simulink model "TADPOLE_Closed_Loop_v2"  (R2024b)
settings: Solver=VariableStepAuto  StartTime=0.0  StopTime=19  RelTol=1e-3
InitFcn:
  | clear mex;
values from neighbouring files (symbols this model uses):
  ipa_tank = 700    [TADPOLEControl.m]
  ox_tank = 600    [TADPOLEControl.m]
  timeDelta = 1/5000    (= 0.0002)    [TADPOLEControl.m]
  timeDeltaCMD = 1/1000    (= 0.001)    [TADPOLEControl.m]
  timeDeltaOUT = 1/200    (= 0.005)    [TADPOLEControl.m]
  x0 = [0 0 0 0]    [TADPOLEControl.m]
undefined symbols (not defined in the file or in its folder): DiscIntNeverNeededParam
settings Model: Creator=pplat  LastModifiedBy=pplat
settings DebuggingCC: AlgebraicLoopMsg=none

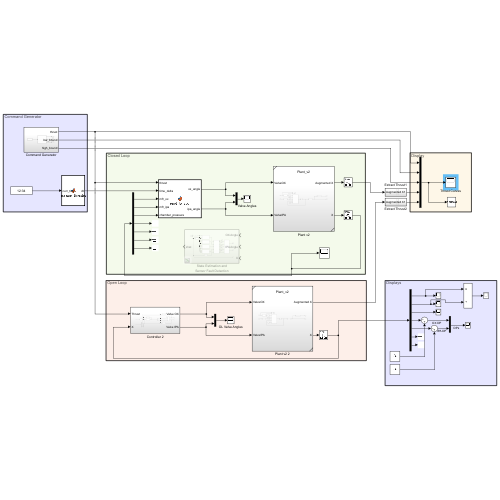
[thumbnail: Simulink's stored preview of the top-level diagram]
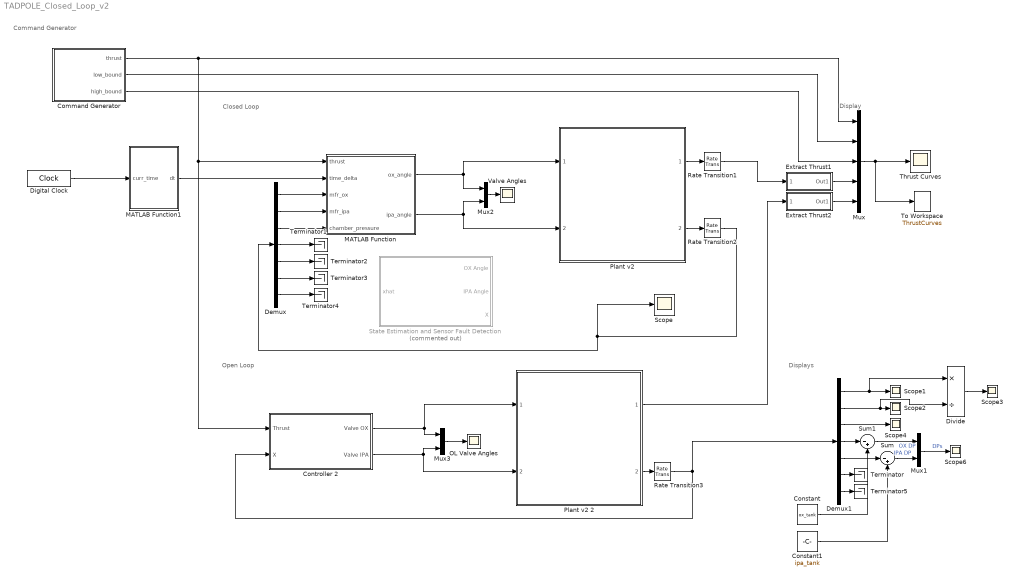
== system TADPOLE_Closed_Loop_v2 ==
  note: Displays
  note: Display
  note: Open Loop
  note: Closed Loop
  note: Command Generator
  Command Generator : Subsystem
  Constant : Constant  Value=ox_tank
  Constant1 : Constant  Value=ipa_tank
  Controller 2 : Subsystem
  Demux : Demux  Outputs=7
  Demux1 : Demux  Outputs=7
  Digital Clock : DigitalClock  SampleTime=timeDelta
  Divide : Product  Inputs=*/
  Extract Thrust1 : Subsystem
  Extract Thrust2 : Subsystem
  MATLAB Function : MATLAB Function  TreatAsAtomicUnit=on
  MATLAB Function1 : MATLAB Function  TreatAsAtomicUnit=on
  Mux : Mux  Inputs=5
  Mux1 : Mux  Inputs=2
  Mux2 : Mux  Inputs=2
  Mux3 : Mux  Inputs=2
  OL Valve Angles : Scope
  Plant v2 : Subsystem  ReferencedSubsystem=Plant_v2
  Plant v2 2 : Subsystem  ReferencedSubsystem=Plant_v2
  Rate Transition1 : RateTransition  OutPortSampleTime=timeDeltaOUT
  Rate Transition2 : RateTransition  OutPortSampleTime=timeDeltaOUT
  Rate Transition3 : RateTransition  OutPortSampleTime=timeDeltaOUT
  Scope{,1..4,6} (6 alike) : Scope
  State Estimation and Sensor Fault Detection : Subsystem  Commented=on
  Sum : Sum  Inputs=|-+
  Sum1 : Sum  Inputs=|-+
  Terminator{,1..5} (6 alike) : Terminator
  Thrust Curves : Scope
  To Workspace : ToWorkspace  VariableName=ThrustCurves  SaveFormat=Timeseries  SampleTime=-1
  Valve Angles : Scope
  wires:
  Mux/1 -> To Workspace/1, Thrust Curves/1
  Mux2/1 -> Valve Angles/1
  Command Generator/1(thrust) -> Mux/1, Controller 2/1(Thrust), MATLAB Function/1(thrust)
  Command Generator/2(low_bound) -> Mux/2
  Command Generator/3(high_bound) -> Mux/3
  MATLAB Function1/1(dt) -> MATLAB Function/2(time_delta)
  Mux3/1 -> OL Valve Angles/1
  Digital Clock/1 -> MATLAB Function1/1(curr_time)
  MATLAB Function/1(ox_angle) -> Mux2/1, Plant v2/1
  MATLAB Function/2(ipa_angle) -> Plant v2/2, Mux2/2
  Controller 2/1(Valve OX) -> Plant v2 2/1, Mux3/1
  Controller 2/2(Valve IPA) -> Plant v2 2/2, Mux3/2
  Extract Thrust1/1(Out1) -> Mux/4
  Extract Thrust2/1(Out1) -> Mux/5
  Plant v2/1 -> Rate Transition1/1
  Plant v2 2/1 -> Extract Thrust2/1(Augmented X)
  Rate Transition1/1 -> Extract Thrust1/1(Augmented X)
  Plant v2/2 -> Rate Transition2/1
  Demux/3 -> MATLAB Function/5(chamber_pressure)
  Demux/2 -> MATLAB Function/4(mfr_ipa)
  Demux/1 -> MATLAB Function/3(mfr_ox)
  Demux/4 -> Terminator1/1
  Demux/5 -> Terminator2/1
  Rate Transition2/1 -> Scope/1, Demux/1
  Demux/6 -> Terminator3/1
  Demux/7 -> Terminator4/1
  Sum1/1 -> Mux1/1  "OX DP"
  Demux1/3 -> Scope4/1
  Divide/1 -> Scope3/1
  Demux1/2 -> Divide/2, Scope2/1
  Mux1/1 -> Scope6/1  "DPs"
  Plant v2 2/2 -> Rate Transition3/1
  Demux1/4 -> Sum1/1
  Demux1/1 -> Divide/1, Scope1/1
  Demux1/5 -> Sum/1
  Constant/1 -> Sum1/2
  Constant1/1 -> Sum/2
  Sum/1 -> Mux1/2  "IPA DP"
  Demux1/6 -> Terminator/1
  Demux1/7 -> Terminator5/1
  Rate Transition3/1 -> Controller 2/2(X), Demux1/1

== system TADPOLE_Closed_Loop_v2/Command Generator ==
  Digital Clock : DigitalClock  SampleTime=timeDelta
  MATLAB Function : MATLAB Function  TreatAsAtomicUnit=on
  thrust : Outport
  low_bound : Outport  Port=2
  high_bound : Outport  Port=3
  wires:
  MATLAB Function/1(thrust) -> thrust/1
  Digital Clock/1 -> MATLAB Function/1(time)
  MATLAB Function/2(low_bound) -> low_bound/1
  MATLAB Function/3(high_bound) -> high_bound/1

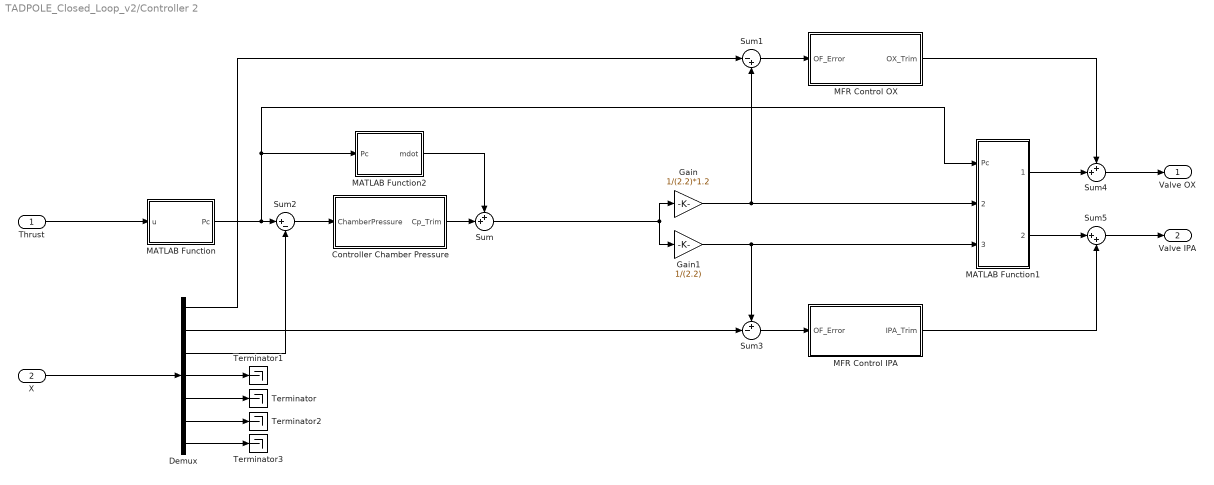
== system TADPOLE_Closed_Loop_v2/Controller 2 ==
  Thrust : Inport
  X : Inport  Port=2
  Controller Chamber Pressure : Subsystem
      settings: PortSchema="{\"entries\":[{\"content\":{\"sides\":[{\"content\":{\"connectorIds\":[\"Out1\"]},\"type\":\"ConnectorPlacement.EquallySpacedRectSide\",\"uuid\":\"33f68c87-1ae2-45d4-8ad9-4cf3c5bc8584\"},{\"content\":{\"connectorIds\":[\"In1\"],\"side\":\"RIGHT\"},\"type\":\"ConnectorPlacement.EquallySpacedRectSide\",\"uuid\":\"17976ab6-0faa-4d7d-91ba-f8a21a62dc32\"},{\"content\":{\"side\":\"TOP\"},\"type\":\"ConnectorPlacement.EquallySpacedRectSide\",\"uuid\":\"89a256ba-7dd2-41f4-a68b-27cc674e20da\"},{\"content\":{\"side\":\"BOTTOM\"},\"type\":\"ConnectorPlacement.EquallySpacedRectSide\",\"uuid\":\"73e60893-e40b-4ea1-8c2d-1d944b0843d3\"}]},\"type\":\"ConnectorPlacement.EquallySpacedConnector\",\"uuid\":\"c17bed4f-f3ae-43fd-abcb-ba9ac56db614\"}],\"packageUris\":[\"http://schema.mathworks.com/mf0/Connector/R2020b\"],\"version\":\"1.0\"}"
  Demux : Demux  Outputs=7
  Gain : Gain  Gain=1/(2.2)*1.2
  Gain1 : Gain  Gain=1/(2.2)
  MATLAB Function : MATLAB Function  TreatAsAtomicUnit=on
  MATLAB Function1 : MATLAB Function  TreatAsAtomicUnit=on
  MATLAB Function2 : MATLAB Function  TreatAsAtomicUnit=on
  MFR Control IPA : Subsystem
      settings: PortSchema="{\"entries\":[{\"content\":{\"sides\":[{\"content\":{\"connectorIds\":[\"Out1\"]},\"type\":\"ConnectorPlacement.EquallySpacedRectSide\",\"uuid\":\"33f68c87-1ae2-45d4-8ad9-4cf3c5bc8584\"},{\"content\":{\"connectorIds\":[\"In1\"],\"side\":\"RIGHT\"},\"type\":\"ConnectorPlacement.EquallySpacedRectSide\",\"uuid\":\"17976ab6-0faa-4d7d-91ba-f8a21a62dc32\"},{\"content\":{\"side\":\"TOP\"},\"type\":\"ConnectorPlacement.EquallySpacedRectSide\",\"uuid\":\"89a256ba-7dd2-41f4-a68b-27cc674e20da\"},{\"content\":{\"side\":\"BOTTOM\"},\"type\":\"ConnectorPlacement.EquallySpacedRectSide\",\"uuid\":\"73e60893-e40b-4ea1-8c2d-1d944b0843d3\"}]},\"type\":\"ConnectorPlacement.EquallySpacedConnector\",\"uuid\":\"c17bed4f-f3ae-43fd-abcb-ba9ac56db614\"}],\"packageUris\":[\"http://schema.mathworks.com/mf0/Connector/R2020b\"],\"version\":\"1.0\"}"
  MFR Control OX : Subsystem
      settings: PortSchema="{\"entries\":[{\"content\":{\"sides\":[{\"content\":{\"connectorIds\":[\"Out1\"]},\"type\":\"ConnectorPlacement.EquallySpacedRectSide\",\"uuid\":\"33f68c87-1ae2-45d4-8ad9-4cf3c5bc8584\"},{\"content\":{\"connectorIds\":[\"In1\"],\"side\":\"RIGHT\"},\"type\":\"ConnectorPlacement.EquallySpacedRectSide\",\"uuid\":\"17976ab6-0faa-4d7d-91ba-f8a21a62dc32\"},{\"content\":{\"side\":\"TOP\"},\"type\":\"ConnectorPlacement.EquallySpacedRectSide\",\"uuid\":\"89a256ba-7dd2-41f4-a68b-27cc674e20da\"},{\"content\":{\"side\":\"BOTTOM\"},\"type\":\"ConnectorPlacement.EquallySpacedRectSide\",\"uuid\":\"73e60893-e40b-4ea1-8c2d-1d944b0843d3\"}]},\"type\":\"ConnectorPlacement.EquallySpacedConnector\",\"uuid\":\"c17bed4f-f3ae-43fd-abcb-ba9ac56db614\"}],\"packageUris\":[\"http://schema.mathworks.com/mf0/Connector/R2020b\"],\"version\":\"1.0\"}"
  Sum : Sum  Inputs=++|
  Sum1 : Sum  Inputs=|-+
  Sum2 : Sum  Inputs=|+-
  Sum3 : Sum  Inputs=+-|
  Sum4 : Sum  Inputs=++|
  Sum5 : Sum  Inputs=|++
  Terminator{,1..3} (4 alike) : Terminator
  Valve OX : Outport
  Valve IPA : Outport  Port=2
  wires:
  MATLAB Function/1(Pc) -> MATLAB Function2/1(Pc), MATLAB Function1/1(Pc), Sum2/1
  MATLAB Function2/1(mdot) -> Sum/1
  Sum2/1 -> Controller Chamber Pressure/1(ChamberPressure)
  Controller Chamber Pressure/1(Cp_Trim) -> Sum/2
  Demux/1 -> Sum1/1
  Demux/2 -> Sum3/2
  Sum3/1 -> MFR Control IPA/1(OF_Error)
  Sum1/1 -> MFR Control OX/1(OF_Error)
  Thrust/1 -> MATLAB Function/1(u)
  Sum/1 -> Gain/1, Gain1/1
  Gain/1 -> Sum1/2, MATLAB Function1/2(mdot_ox)
  Gain1/1 -> MATLAB Function1/3(mdot_ipa), Sum3/1
  X/1 -> Demux/1
  Demux/5 -> Terminator/1
  Demux/4 -> Terminator1/1
  Demux/3 -> Sum2/2
  Sum5/1 -> Valve IPA/1
  MATLAB Function1/2(theta_ipa) -> Sum5/1
  MATLAB Function1/1(theta_ox) -> Sum4/2
  Sum4/1 -> Valve OX/1
  MFR Control OX/1(OX_Trim) -> Sum4/1
  MFR Control IPA/1(IPA_Trim) -> Sum5/2
  Demux/6 -> Terminator2/1
  Demux/7 -> Terminator3/1

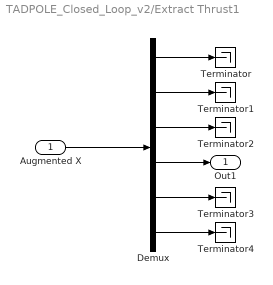
== system TADPOLE_Closed_Loop_v2/Extract Thrust1 ==
  Augmented X : Inport
  Demux : Demux  Outputs=6
  Terminator{,1..4} (5 alike) : Terminator
  Out1 : Outport
  wires:
  Augmented X/1 -> Demux/1
  Demux/1 -> Terminator/1
  Demux/2 -> Terminator1/1
  Demux/3 -> Terminator2/1
  Demux/5 -> Terminator3/1
  Demux/6 -> Terminator4/1
  Demux/4 -> Out1/1

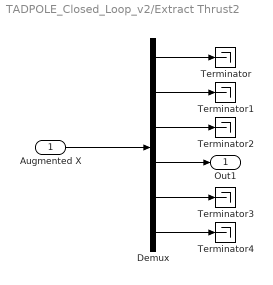
== system TADPOLE_Closed_Loop_v2/Extract Thrust2 ==
  Augmented X : Inport
  Demux : Demux  Outputs=6
  Terminator{,1..4} (5 alike) : Terminator
  Out1 : Outport
  wires:
  Augmented X/1 -> Demux/1
  Demux/1 -> Terminator/1
  Demux/2 -> Terminator1/1
  Demux/3 -> Terminator2/1
  Demux/5 -> Terminator3/1
  Demux/6 -> Terminator4/1
  Demux/4 -> Out1/1

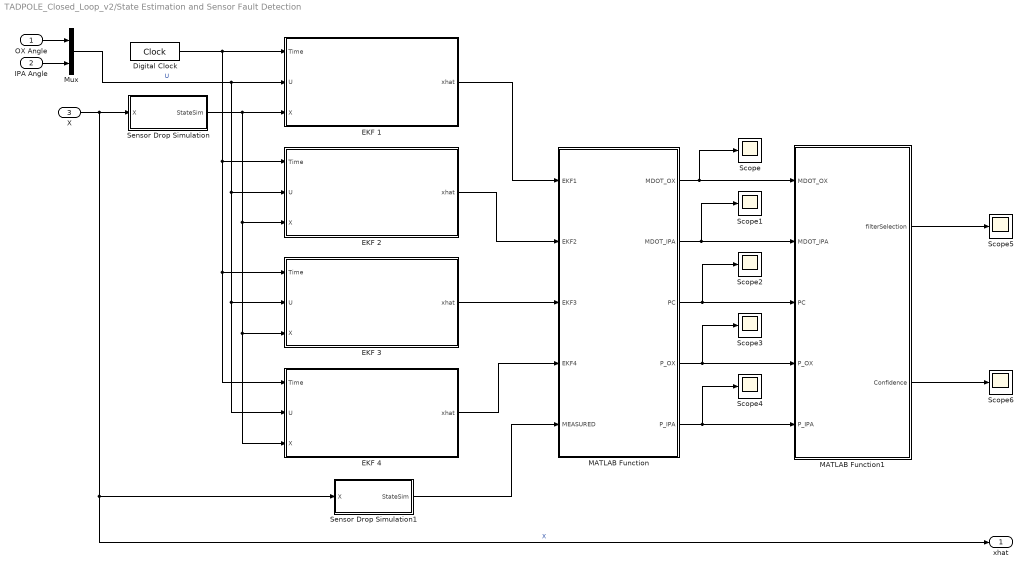
== system TADPOLE_Closed_Loop_v2/State Estimation and Sensor Fault Detection ==
  OX Angle : Inport
  IPA Angle : Inport  Port=2
  X : Inport  Port=3
  Digital Clock : DigitalClock  SampleTime=timeDeltaOUT
  EKF 1 : Subsystem
  EKF 2 : Subsystem
  EKF 3 : Subsystem
  EKF 4 : Subsystem
  MATLAB Function : MATLAB Function  TreatAsAtomicUnit=on
  MATLAB Function1 : MATLAB Function  TreatAsAtomicUnit=on
  Mux : Mux  Inputs=2
  Scope{,1..6} (7 alike) : Scope
  Sensor Drop Simulation : Subsystem
  Sensor Drop Simulation1 : Subsystem
  xhat : Outport
  wires:
  IPA Angle/1 -> Mux/2
  OX Angle/1 -> Mux/1
  X/1 -> Sensor Drop Simulation/1(X), xhat/1, Sensor Drop Simulation1/1(X)  "X"
  Mux/1 -> EKF 3/2(U), EKF 4/2(U), EKF 2/2(U), EKF 1/2(U)  "U"
  Digital Clock/1 -> EKF 3/1(Time), EKF 4/1(Time), EKF 2/1(Time), EKF 1/1(Time)
  Sensor Drop Simulation/1(StateSim) -> EKF 2/3(X), EKF 3/3(X), EKF 4/3(X), EKF 1/3(X)
  EKF 1/1(xhat) -> MATLAB Function/1(EKF1)
  EKF 2/1(xhat) -> MATLAB Function/2(EKF2)
  EKF 3/1(xhat) -> MATLAB Function/3(EKF3)
  EKF 4/1(xhat) -> MATLAB Function/4(EKF4)
  Sensor Drop Simulation1/1(StateSim) -> MATLAB Function/5(MEASURED)
  MATLAB Function/5(P_IPA) -> MATLAB Function1/5(P_IPA), Scope4/1
  MATLAB Function/4(P_OX) -> MATLAB Function1/4(P_OX), Scope3/1
  MATLAB Function/3(PC) -> Scope2/1, MATLAB Function1/3(PC)
  MATLAB Function/2(MDOT_IPA) -> MATLAB Function1/2(MDOT_IPA), Scope1/1
  MATLAB Function/1(MDOT_OX) -> Scope/1, MATLAB Function1/1(MDOT_OX)
  MATLAB Function1/1(filterSelection) -> Scope5/1
  MATLAB Function1/2(Confidence) -> Scope6/1

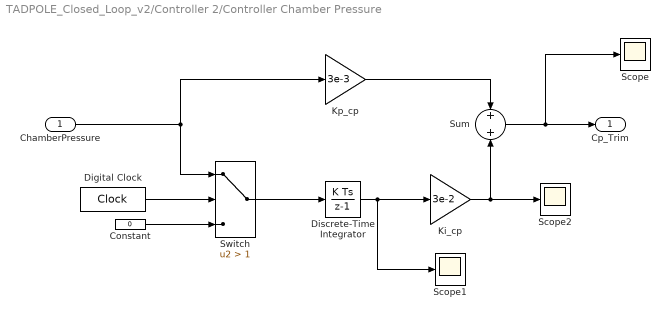
== system TADPOLE_Closed_Loop_v2/Controller 2/Controller Chamber Pressure ==
  ChamberPressure : Inport
  Constant : Constant  Value=0
  Digital Clock : DigitalClock  SampleTime=timeDeltaCMD
  Discrete-Time Integrator : DiscreteIntegrator  SampleTime=-1  ICPrevOutput=DiscIntNeverNeededParam  ICPrevScaledInput=DiscIntNeverNeededParam
  Ki_cp : Gain  Gain=3e-2
  Kp_cp : Gain  Gain=3e-3
  Scope : Scope
  Scope1 : Scope
  Scope2 : Scope
  Sum : Sum  Inputs=+|+
  Switch : Switch  Criteria=u2 > Threshold  Threshold=1  SaturateOnIntegerOverflow=off  InputSameDT=off
  Cp_Trim : Outport
  wires:
  Kp_cp/1 -> Sum/1
  Discrete-Time Integrator/1 -> Scope1/1, Ki_cp/1
  ChamberPressure/1 -> Switch/1, Kp_cp/1
  Sum/1 -> Scope/1, Cp_Trim/1
  Digital Clock/1 -> Switch/2
  Switch/1 -> Discrete-Time Integrator/1
  Constant/1 -> Switch/3
  Ki_cp/1 -> Scope2/1, Sum/2

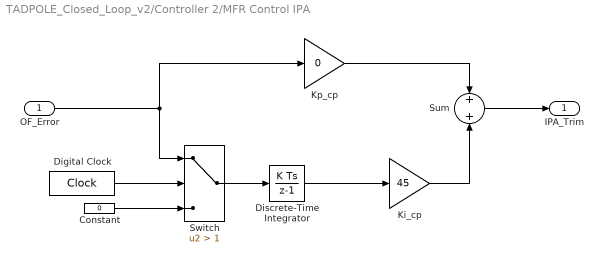
== system TADPOLE_Closed_Loop_v2/Controller 2/MFR Control IPA ==
  OF_Error : Inport
  Constant : Constant  Value=0
  Digital Clock : DigitalClock  SampleTime=timeDeltaCMD
  Discrete-Time Integrator : DiscreteIntegrator  SampleTime=-1  ICPrevOutput=DiscIntNeverNeededParam  ICPrevScaledInput=DiscIntNeverNeededParam
  Ki_cp : Gain  Gain=45
  Kp_cp : Gain  Gain=0
  Sum : Sum  Inputs=+|+
  Switch : Switch  Criteria=u2 > Threshold  Threshold=1  SaturateOnIntegerOverflow=off  InputSameDT=off
  IPA_Trim : Outport
  wires:
  Discrete-Time Integrator/1 -> Ki_cp/1
  Sum/1 -> IPA_Trim/1
  Ki_cp/1 -> Sum/2
  Kp_cp/1 -> Sum/1
  Constant/1 -> Switch/3
  Digital Clock/1 -> Switch/2
  OF_Error/1 -> Switch/1, Kp_cp/1
  Switch/1 -> Discrete-Time Integrator/1

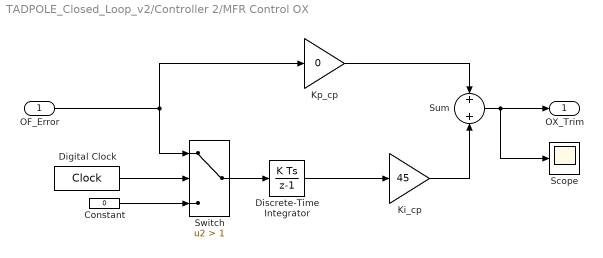
== system TADPOLE_Closed_Loop_v2/Controller 2/MFR Control OX ==
  OF_Error : Inport
  Constant : Constant  Value=0
  Digital Clock : DigitalClock  SampleTime=timeDeltaCMD
  Discrete-Time Integrator : DiscreteIntegrator  SampleTime=-1  ICPrevOutput=DiscIntNeverNeededParam  ICPrevScaledInput=DiscIntNeverNeededParam
  Ki_cp : Gain  Gain=45
  Kp_cp : Gain  Gain=0
  Scope : Scope
  Sum : Sum  Inputs=+|+
  Switch : Switch  Criteria=u2 > Threshold  Threshold=1  SaturateOnIntegerOverflow=off  InputSameDT=off
  OX_Trim : Outport
  wires:
  Discrete-Time Integrator/1 -> Ki_cp/1
  Sum/1 -> Scope/1, OX_Trim/1
  Ki_cp/1 -> Sum/2
  Kp_cp/1 -> Sum/1
  Constant/1 -> Switch/3
  Digital Clock/1 -> Switch/2
  OF_Error/1 -> Switch/1, Kp_cp/1
  Switch/1 -> Discrete-Time Integrator/1

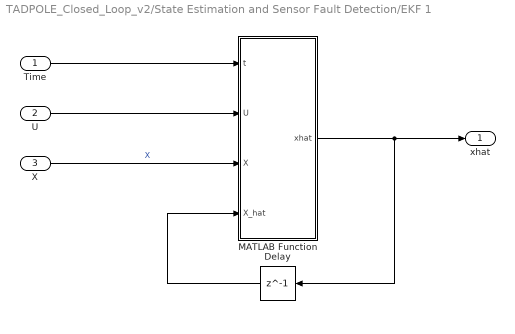
== system TADPOLE_Closed_Loop_v2/State Estimation and Sensor Fault Detection/EKF 1 ==
  Time : Inport
  U : Inport  Port=2
  X : Inport  Port=3
  Delay : Delay  DelayLength=1  InitialCondition=x0.'
  MATLAB Function : MATLAB Function  TreatAsAtomicUnit=on
  xhat : Outport
  wires:
  Time/1 -> MATLAB Function/1(t)
  Delay/1 -> MATLAB Function/4(X_hat)
  MATLAB Function/1(xhat) -> xhat/1, Delay/1
  X/1 -> MATLAB Function/3(X)  "X"
  U/1 -> MATLAB Function/2(U)

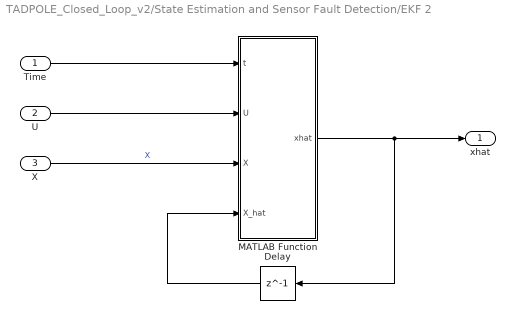
== system TADPOLE_Closed_Loop_v2/State Estimation and Sensor Fault Detection/EKF 2 ==
  Time : Inport
  U : Inport  Port=2
  X : Inport  Port=3
  Delay : Delay  DelayLength=1  InitialCondition=x0.'
  MATLAB Function : MATLAB Function  TreatAsAtomicUnit=on
  xhat : Outport
  wires:
  Time/1 -> MATLAB Function/1(t)
  Delay/1 -> MATLAB Function/4(X_hat)
  MATLAB Function/1(xhat) -> xhat/1, Delay/1
  X/1 -> MATLAB Function/3(X)  "X"
  U/1 -> MATLAB Function/2(U)

== system TADPOLE_Closed_Loop_v2/State Estimation and Sensor Fault Detection/EKF 3 ==
  Time : Inport
  U : Inport  Port=2
  X : Inport  Port=3
  Delay : Delay  DelayLength=1  InitialCondition=x0.'
  MATLAB Function : MATLAB Function  TreatAsAtomicUnit=on
  xhat : Outport
  wires:
  Time/1 -> MATLAB Function/1(t)
  Delay/1 -> MATLAB Function/4(X_hat)
  MATLAB Function/1(xhat) -> xhat/1, Delay/1
  X/1 -> MATLAB Function/3(X)  "X"
  U/1 -> MATLAB Function/2(U)

== system TADPOLE_Closed_Loop_v2/State Estimation and Sensor Fault Detection/EKF 4 ==
  Time : Inport
  U : Inport  Port=2
  X : Inport  Port=3
  Delay : Delay  DelayLength=1  InitialCondition=x0.'
  MATLAB Function : MATLAB Function  TreatAsAtomicUnit=on
  xhat : Outport
  wires:
  Time/1 -> MATLAB Function/1(t)
  Delay/1 -> MATLAB Function/4(X_hat)
  MATLAB Function/1(xhat) -> xhat/1, Delay/1
  X/1 -> MATLAB Function/3(X)  "X"
  U/1 -> MATLAB Function/2(U)

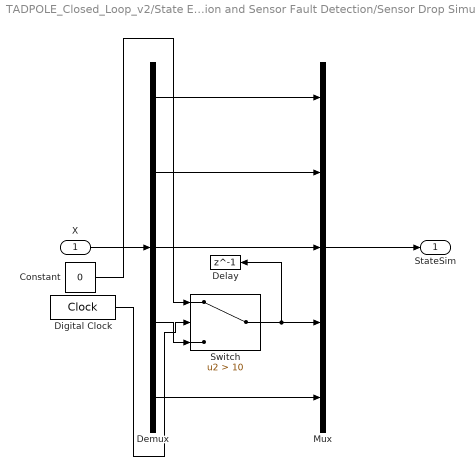
== system TADPOLE_Closed_Loop_v2/State Estimation and Sensor Fault Detection/Sensor Drop Simulation ==
  X : Inport
  Constant : Constant  Value=0
  Delay : Delay  DelayLength=1
  Demux : Demux  Outputs=5
  Digital Clock : DigitalClock  SampleTime=timeDeltaOUT
  Mux : Mux  Inputs=5
  Switch : Switch  Criteria=u2 > Threshold  Threshold=10  SaturateOnIntegerOverflow=off  InputSameDT=off
  StateSim : Outport
  wires:
  X/1 -> Demux/1
  Mux/1 -> StateSim/1
  Demux/1 -> Mux/1
  Demux/2 -> Mux/2
  Demux/3 -> Mux/3
  Demux/5 -> Mux/5
  Digital Clock/1 -> Switch/2
  Switch/1 -> Delay/1, Mux/4
  Demux/4 -> Switch/3
  Constant/1 -> Switch/1

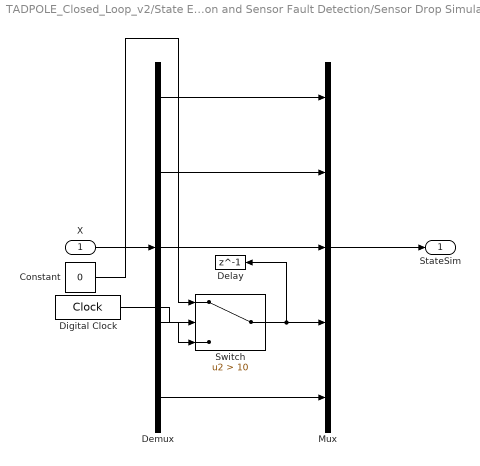
== system TADPOLE_Closed_Loop_v2/State Estimation and Sensor Fault Detection/Sensor Drop Simulation1 ==
  X : Inport
  Constant : Constant  Value=0
  Delay : Delay  DelayLength=1
  Demux : Demux  Outputs=5
  Digital Clock : DigitalClock  SampleTime=timeDeltaOUT
  Mux : Mux  Inputs=5
  Switch : Switch  Criteria=u2 > Threshold  Threshold=10  SaturateOnIntegerOverflow=off  InputSameDT=off
  StateSim : Outport
  wires:
  X/1 -> Demux/1
  Mux/1 -> StateSim/1
  Demux/1 -> Mux/1
  Demux/2 -> Mux/2
  Demux/3 -> Mux/3
  Demux/5 -> Mux/5
  Digital Clock/1 -> Switch/2
  Switch/1 -> Delay/1, Mux/4
  Demux/4 -> Switch/3
  Constant/1 -> Switch/1

== matlab function TADPOLE_Closed_Loop_v2/Controller 2/MATLAB Function ==
  data: u input; Pc output
function Pc = T2PC(u)

    Pc = thrust_to_cp(u);
end

== matlab function TADPOLE_Closed_Loop_v2/Controller 2/MATLAB Function1 ==
  data: Pc input; mdot_ox input; mdot_ipa input; theta_ox output; theta_ipa output
function [theta_ox, theta_ipa] = angles(Pc, mdot_ox, mdot_ipa)

    [theta_ox, theta_ipa] = mdot2valves(mdot_ox, mdot_ipa, Pc);
end

== matlab function TADPOLE_Closed_Loop_v2/Controller 2/MATLAB Function2 ==
  data: Pc input; mdot output
function mdot = PC2MDOT(Pc)

    mdot = 1.69 * Pc / fcn_cstar(1.2, Pc) * 32.174;
end

== matlab function TADPOLE_Closed_Loop_v2/MATLAB Function ==
  data: thrust input; time_delta input; ox_angle output; ipa_angle output; mfr_ox input; mfr_ipa input; chamber_pressure input
function [ox_angle, ipa_angle] = send_to_cpp(thrust, time_delta, mfr_ox, mfr_ipa, chamber_pressure)
coder.extrinsic('closed_loop_valve_control_wrap');  % Declare MEX function as extrinsic
ox_angle = 0;
ipa_angle = 0;
[ox_angle, ipa_angle] = closed_loop_valve_control_wrap(thrust, time_delta, mfr_ox, mfr_ipa, chamber_pressure);

== matlab function TADPOLE_Closed_Loop_v2/MATLAB Function1 ==
  data: dt output; curr_time input
function dt = measure_timestep(curr_time)
    persistent prev_time;
    if isempty(prev_time)
        prev_time = 0;
    end
    if curr_time < 0.3
        dt = 0;
    else
        dt = curr_time - prev_time;
    end
    prev_time = curr_time;
end

== matlab function TADPOLE_Closed_Loop_v2/Command Generator/MATLAB Function ==
  data: time input; thrust output; low_bound output; high_bound output
function [thrust,low_bound,high_bound] = thrustCurveBounds(time)
thrust = holdT(time);
t_past = holdT(time - 0.5);
t_future = holdT(time + 0.5);

high_bound = max([thrust, t_past, t_future]) + 0.05 * 550;
low_bound = min([thrust, t_past, t_future]) - 0.05 * 550;

end

== matlab function TADPOLE_Closed_Loop_v2/State Estimation and Sensor Fault Detection/EKF 2/MATLAB Function ==
  data: t input; U input; X input; xhat output; X_hat input
function xhat = Estimate(t, U, X, X_hat)

    C = [0 0 0 1 0;
         0 0 0 0 1];
    
    xhat = EstimateState(X, X_hat, U, t, C);
end

== matlab function TADPOLE_Closed_Loop_v2/State Estimation and Sensor Fault Detection/EKF 1/MATLAB Function ==
  data: t input; U input; X input; xhat output; X_hat input
function xhat = Estimate(t, U, X, X_hat)

    C = [0 0 1 0 0;
         0 0 0 1 0;
         0 0 0 0 1];
    
    xhat = EstimateState(X, X_hat, U, t, C);
end

== matlab function TADPOLE_Closed_Loop_v2/State Estimation and Sensor Fault Detection/EKF 3/MATLAB Function ==
  data: t input; U input; X input; xhat output; X_hat input
function xhat = Estimate(t, U, X, X_hat)

    C = [0 0 1 0 0;
         0 0 0 0 1];
    
    xhat = EstimateState(X, X_hat, U, t, C);
end

== matlab function TADPOLE_Closed_Loop_v2/State Estimation and Sensor Fault Detection/EKF 4/MATLAB Function ==
  data: t input; U input; X input; xhat output; X_hat input
function xhat = Estimate(t, U, X, X_hat)

    C = [0 0 1 0 0;
         0 0 0 1 0];
    
    xhat = EstimateState(X, X_hat, U, t, C);
end

== matlab function TADPOLE_Closed_Loop_v2/State Estimation and Sensor Fault Detection/MATLAB Function ==
  data: EKF1 input; MDOT_OX output; EKF2 input; EKF3 input; EKF4 input; MEASURED input; MDOT_IPA output; PC output; P_OX output; P_IPA output
function [MDOT_OX, MDOT_IPA, PC, P_OX, P_IPA] = extractStates(EKF1, EKF2, EKF3, EKF4, MEASURED)

    MDOT_OX = [EKF1(1); EKF2(1); EKF3(1); EKF4(1); MEASURED(1)];
    MDOT_IPA = [EKF1(2); EKF2(2); EKF3(2); EKF4(2); MEASURED(2)];
    PC = [EKF1(3); EKF2(3); EKF3(3); EKF4(3); MEASURED(3)];
    P_OX = [EKF1(4); EKF2(4); EKF3(4); EKF4(4); MEASURED(4)];
    P_IPA = [EKF1(5); EKF2(5); EKF3(5); EKF4(5); MEASURED(5)];

end

== matlab function TADPOLE_Closed_Loop_v2/State Estimation and Sensor Fault Detection/MATLAB Function1 ==
  data: MDOT_OX input; filterSelection output; MDOT_IPA input; PC input; P_OX input; P_IPA input; Confidence output
function [filterSelection, Confidence] = Select(MDOT_OX, MDOT_IPA, PC, P_OX, P_IPA)
    
    [filterSelection, Confidence] = filterSelect(MDOT_OX, MDOT_IPA, PC, P_OX, P_IPA);
end
